simulink model "wheelchair_navigation"  (R2025b)
settings: Solver=VariableStepAuto  StartTime=0.0  StopTime=30  FixedStep=Ts  MaxStep=1.0  RelTol=1e-3
model workspace: external: MAT-File (data not in the file)
values from neighbouring files (symbols this model uses):
  a_max = 0.20    (= 0.2)    [init.m]
  AMCL_param = [rho,m_pos,q_pos,m_theta,q_theta,sigma_min_fact,sigma_max_fact,     p_fail,lost_duration,qt_lost_thd,max_jump_dist]    [init.m]
  d = 0.650    (= 0.65)    [init.m]
  e = 0.1    [init.m]
  epsilon = 0.5    [init.m]
  N = 20    [init.m]
  N_samples = 40    [init.m]
  omega_M = v_max/Rw    (= 1.52777777778)    [init.m]
  omega_m = -v_max/Rw    (= -1.52777777778)    [init.m]
  pos_estim_param = [sigma_q,sigma_m]    [init.m]
  q = 1    [init.m]
  r = 1    [init.m]
  r_c = 0.75    [init.m]
  r_red = 0.3    [init.m]
  Rw = 0.36    [init.m]
  s = (q+k^2*r)/(1-(1+Ts*k)^2)    (= 9.66666666667)    [init.m]
  sa = 10^3    (= 1000)    [init.m]
  sp = 10^9    (= 1000000000)    [init.m]
  T_gp = 4    [init.m]
  Ts = 0.2    [init.m]
  Ts_pedpos_est = 0.1    [init.m]
  v_max = 0.55    [init.m]
  x_p0 = startLoc(1)    [init.m]
  y_p0 = startLoc(2)    [init.m]
undefined symbols (not defined in the file or in its folder): endLoc, initial_cond, n_obs, param, Ped_init, qd, qdd, v_ped, v_ped_fun, x_pri, y_pri
libraries: simulink x1
settings Model: PacingRate=5  Creator=Lenovo ThinkPad  LastModifiedBy=bascetta
settings SolverCC: AlgebraicLoopSolver=TrustRegion
settings DataIOCC: SaveOutput=off  SignalLogging=off  DSMLogging=off  SaveTime=off  ReturnWorkspaceOutputs=off
settings OptimizationCC: ReuseModelBlockBuffer=off
settings DebuggingCC: UnconnectedInputMsg=warning  UnconnectedOutputMsg=warning  UnconnectedLineMsg=warning  UnderSpecifiedDimensionMsg=warning
settings ModelReferenceCC: EnableRefExpFcnMdlSchedulingChecks=on
settings SFSimCC: CustomCodeUndefinedFunction=UseInterfaceOnly
settings RTWCC: GPUComputeCapability=3.5  DLArmComputeVersion=19.05

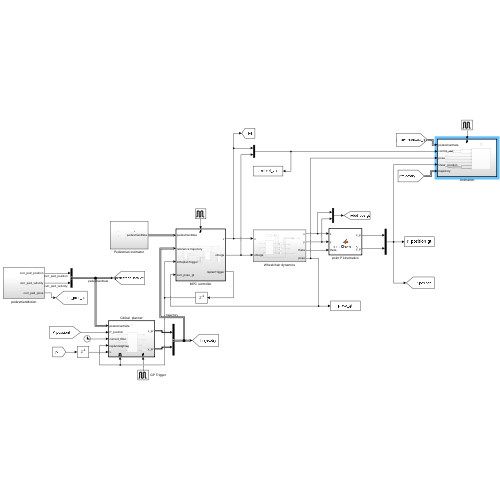
[thumbnail: Simulink's stored preview of the top-level diagram]
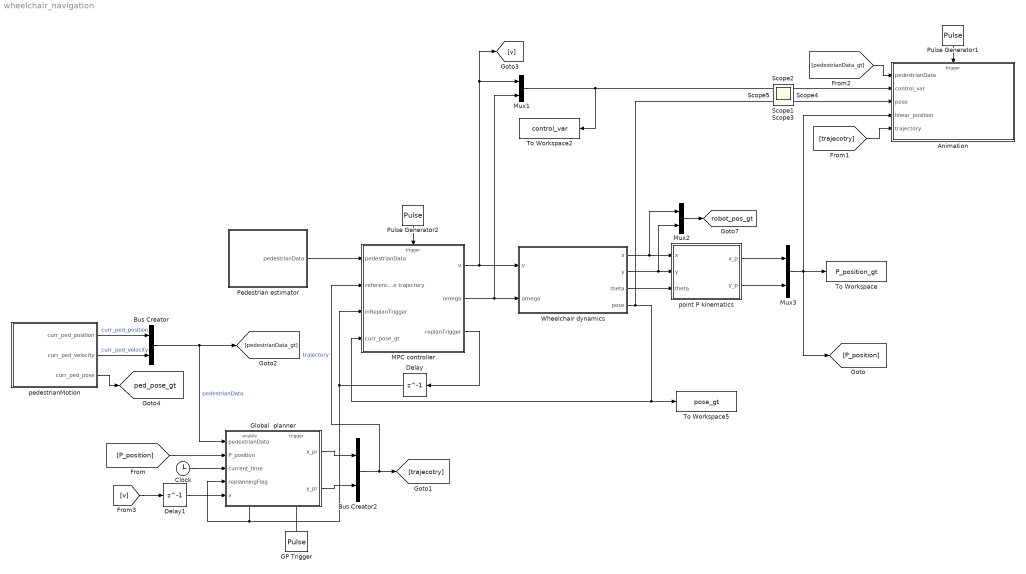
== system wheelchair_navigation ==
  Animation : Subsystem
  Bus Creator : BusCreator  Inputs=2
  Bus Creator2 : BusCreator  Inputs=2
  Clock : Clock
  Delay : Delay  DelayLength=1  InitialCondition=1  SampleTime=Ts
  Delay1 : Delay  DelayLength=1  InitialCondition=0  SampleTime=Ts
  GP Trigger : DiscretePulseGenerator  PulseType=Time based  Period=T_gp  PulseWidth=50  PhaseDelay=1e-16
  Global  planner : Subsystem
  MPC controller : Subsystem  TreatAsAtomicUnit=on
  Mux1 : Mux  Inputs=2
  Mux2 : Mux  Inputs=2
  Mux3 : Mux  Inputs=2
  Pedestrian estimator : Subsystem
  Pulse Generator1 : DiscretePulseGenerator  PulseType=Time based  Period=Ts  PulseWidth=50  PhaseDelay=1e-16
  Pulse Generator2 : DiscretePulseGenerator  PulseType=Time based  Period=Ts  PulseWidth=50  PhaseDelay=1e-16
  To Workspace : ToWorkspace  VariableName=P_position_gt  SaveFormat=Structure With Time  SampleTime=Ts
  To Workspace2 : ToWorkspace  VariableName=control_var  SaveFormat=Structure With Time  SampleTime=Ts
  To Workspace5 : ToWorkspace  VariableName=pose_gt  SaveFormat=Structure With Time  SampleTime=Ts
  "Wheelchair dynamics " : Subsystem
  pedestrianMotion : Subsystem
  point P kinematics : MATLAB Function  TreatAsAtomicUnit=on
  Scope{1..5} (5 alike) : Scope
      Scope1 settings: ActiveDisplayYMinimum=-0.0525  ActiveDisplayYMaximum=0.4725  DataLoggingVariableName=ScopeData3
      Scope3 settings: ActiveDisplayYMinimum=-0.13667  ActiveDisplayYMaximum=1.23002  DataLoggingVariableName=ScopeData2
      Scope5 settings: DataLoggingVariableName=ScopeData2
  tag scope: ped_pose_gt=global, robot_pos_gt=global
  wires:
  Pulse Generator2/1 -> MPC controller/Trigger
  "Wheelchair dynamics "/1(x) -> Mux2/1, point P kinematics/1(x)
  "Wheelchair dynamics "/2(y) -> Mux2/2, point P kinematics/2(y)
  "Wheelchair dynamics "/3(theta) -> point P kinematics/3(theta)
  MPC controller/1(v) -> [v], Mux1/1, "Wheelchair dynamics "/1(v)
  MPC controller/2(omega) -> Mux1/2, "Wheelchair dynamics "/2(omega)
  Mux1/1 -> To Workspace2/1, Animation/2(control_var)
  point P kinematics/1(x_p) -> Mux3/1
  point P kinematics/2(y_p) -> Mux3/2
  Pulse Generator1/1 -> Animation/Trigger
  Bus Creator/1 -> [pedestrianData_gt], Global  planner/1(pedestrianData)  "pedestrianData"
  pedestrianMotion/2(curr_ped_velocity) -> Bus Creator/2  "curr_ped_velocity"
  pedestrianMotion/1(curr_ped_position) -> Bus Creator/1  "curr_ped_position"
  [P_position] -> Global  planner/2(P_position)
  Clock/1 -> Global  planner/3(current_time)
  Global  planner/1(x_pr) -> Bus Creator2/1
  Global  planner/2(y_pr) -> Bus Creator2/2
  Bus Creator2/1 -> MPC controller/2(reference trajectory), [trajecotry]  "trajectory"
  [trajecotry] -> Animation/5(trajectory)
  [pedestrianData_gt] -> Animation/1(pedestrianData)
  MPC controller/3(replanTrigger) -> Delay/1
  Delay/1 -> Global  planner/4(replanningFlag), Global  planner/Enable, MPC controller/3(inReplanTrigger)
  Mux3/1 -> Animation/4(linear_position), To Workspace/1, [P_position]
  GP Trigger/1 -> Global  planner/Trigger
  [v] -> Delay1/1
  Delay1/1 -> Global  planner/5(v)
  pedestrianMotion/3(curr_ped_pose) -> [ped_pose_gt]
  Mux2/1 -> [robot_pos_gt]
  Pedestrian estimator/1(pedestrianData) -> MPC controller/1(pedestrianData)
  "Wheelchair dynamics "/4(pose) -> Animation/3(pose), To Workspace5/1, MPC controller/4("curr_pose_gt ")

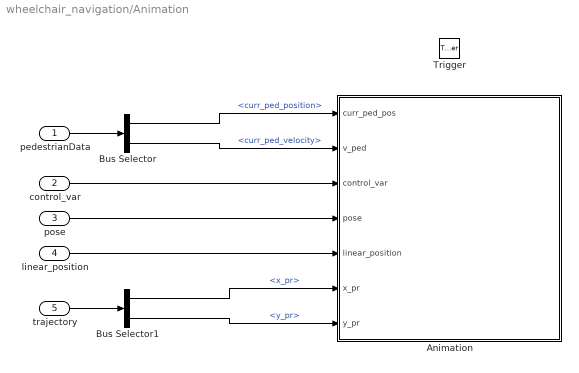
== system wheelchair_navigation/Animation ==
  pedestrianData : Inport
  control_var : Inport  Port=2
  pose : Inport  Port=3
  linear_position : Inport  Port=4
  trajectory : Inport  Port=5
  Trigger : TriggerPort  VariantControl=Variant  PortDimensions=1
  "Animation " : MATLAB Function  TreatAsAtomicUnit=on
  Bus Selector : BusSelector  OutputSignals=curr_ped_position,curr_ped_velocity
  Bus Selector1 : BusSelector  OutputSignals=x_pr,y_pr
  wires:
  pose/1 -> "Animation "/4(pose)
  control_var/1 -> "Animation "/3(control_var)
  linear_position/1 -> "Animation "/5(linear_position)
  pedestrianData/1 -> Bus Selector/1
  Bus Selector/1 -> "Animation "/1(curr_ped_pos)  "<curr_ped_position>"
  Bus Selector/2 -> "Animation "/2(v_ped)  "<curr_ped_velocity>"
  trajectory/1 -> Bus Selector1/1
  Bus Selector1/1 -> "Animation "/6(x_pr)  "<x_pr>"
  Bus Selector1/2 -> "Animation "/7(y_pr)  "<y_pr>"

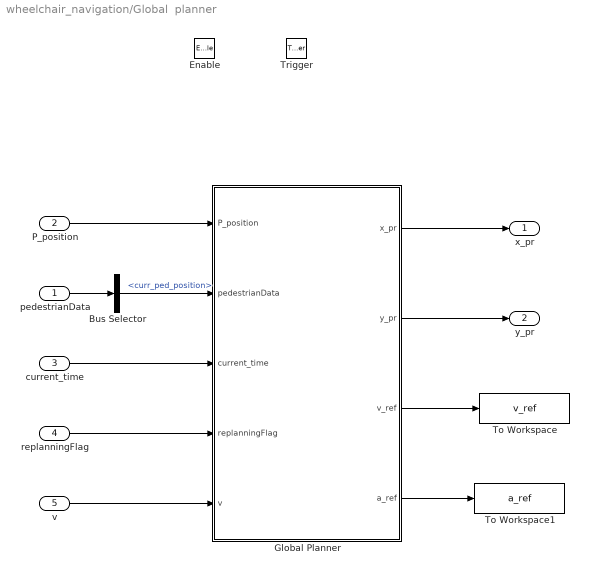
== system wheelchair_navigation/Global  planner ==
  pedestrianData : Inport
  P_position : Inport  Port=2
  current_time : Inport  Port=3
  replanningFlag : Inport  Port=4
  v : Inport  Port=5
  Enable : EnablePort  PropagateVarSize=During execution
  Trigger : TriggerPort  VariantControl=(inherit)  PortDimensions=1
  Bus Selector : BusSelector  OutputSignals=curr_ped_position
  Global Planner : MATLAB Function  TreatAsAtomicUnit=on
  To Workspace : ToWorkspace  VariableName=v_ref  SaveFormat=Timeseries  SampleTime=-1
  To Workspace1 : ToWorkspace  VariableName=a_ref  SaveFormat=Timeseries  SampleTime=-1
  x_pr : Outport
  y_pr : Outport  Port=2
  wires:
  current_time/1 -> Global Planner/3(current_time)
  Bus Selector/1 -> Global Planner/2(pedestrianData)  "<curr_ped_position>"
  pedestrianData/1 -> Bus Selector/1
  Global Planner/1(x_pr) -> x_pr/1
  Global Planner/2(y_pr) -> y_pr/1
  P_position/1 -> Global Planner/1(P_position)
  replanningFlag/1 -> Global Planner/4(replanningFlag)
  v/1 -> Global Planner/5(v)
  Global Planner/3(v_ref) -> To Workspace/1
  Global Planner/4(a_ref) -> To Workspace1/1

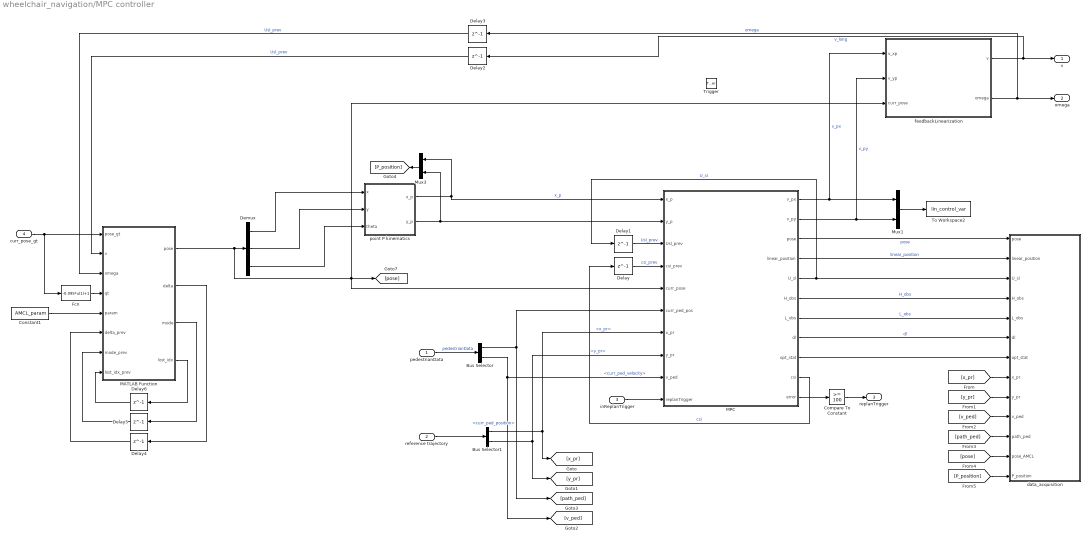
== system wheelchair_navigation/MPC controller ==
  pedestrianData : Inport
  reference trajectory : Inport  Port=2
  inReplanTrigger : Inport  Port=3
  "curr_pose_gt " : Inport  Port=4
  Trigger : TriggerPort  VariantControl=Variant
  Bus Selector : BusSelector  OutputSignals=curr_ped_position,curr_ped_velocity
  Bus Selector1 : BusSelector  OutputSignals=x_pr,y_pr
  Compare To Constant : simulink/Logic and Bit Operations/Compare To Constant  relop=>=  const=100  OutDataTypeStr=boolean
  Constant1 : Constant  Value=AMCL_param
  Delay : Delay  DelayLength=1  InitialCondition=[x_p0;y_p0]
  Delay1 : Delay  DelayLength=1  InitialCondition=0
  Delay2 : Delay  DelayLength=1  InitialCondition=0
  Delay3 : Delay  DelayLength=1  InitialCondition=0
  Delay4 : Delay  DelayLength=1
  Delay5 : Delay  DelayLength=1  InitialCondition=1.0
  Delay6 : Delay  DelayLength=1  InitialCondition=1.0
  Demux : Demux  Outputs=3
  Fcn : Fcn  Expr=-0.095*u(1)+1
  MATLAB Function : MATLAB Function  TreatAsAtomicUnit=on
  MPC : MATLAB Function  TreatAsAtomicUnit=on  mask{Ts=Ts, N=N, v_max=v_max, a_max=a_max, q=q, r=r, d=d, radius=Rw, max_omega=omega_M, min_omega=omega_m, epsilon=epsilon, n_obs=n_obs, e=e, N_samples=N_samples}
  Mux1 : Mux  Inputs=2
  Mux3 : Mux  Inputs=2
  To Workspace2 : ToWorkspace  VariableName=lin_control_var  SaveFormat=Structure With Time  SampleTime=-1
  data_acquisition : Subsystem
  feedbackLinearization : MATLAB Function  TreatAsAtomicUnit=on
  point P kinematics : MATLAB Function  TreatAsAtomicUnit=on
  v : Outport
  omega : Outport  Port=2
  replanTrigger : Outport  Port=3
  wires:
  Delay1/1 -> MPC/3(Usl_prev)  "Usl_prev"
  Delay/1 -> MPC/4(csi_prev)  "csi_prev"
  MPC/3(pose) -> data_acquisition/1(pose)  "pose"
  MPC/4(linear_position) -> data_acquisition/2(linear_position)  "linear_position"
  MPC/5(U_sl) -> Delay1/1, data_acquisition/3(U_sl)  "U_sl"
  MPC/6(H_obs) -> data_acquisition/4("H_obs ")  "H_obs"
  MPC/7(L_obs) -> data_acquisition/5("L_obs ")  "L_obs"
  MPC/8(dl) -> data_acquisition/6(dl)  "dl"
  MPC/10(csi) -> Delay/1  "csi"
  MPC/9(opt_stat) -> data_acquisition/7(opt_stat)
  MPC/1(v_px) -> Mux1/1, feedbackLinearization/1(v_xp)  "v_px"
  MPC/2(v_py) -> Mux1/2, feedbackLinearization/2(v_yp)  "v_py"
  Bus Selector/2 -> [v_ped], MPC/9(v_ped)  "<curr_ped_velocity>"
  pedestrianData/1 -> Bus Selector/1  "pedestrianData"
  Bus Selector/1 -> [path_ped], MPC/6(curr_ped_pos)  "<curr_ped_position>"
  Bus Selector1/1 -> [x_pr], MPC/7(x_pr)  "<x_pr>"
  Bus Selector1/2 -> [y_pr], MPC/8(y_pr)  "<y_pr>"
  reference trajectory/1 -> Bus Selector1/1
  MPC/11(error) -> Compare To Constant/1
  Compare To Constant/1 -> replanTrigger/1
  inReplanTrigger/1 -> MPC/10(replanTrigger)
  [x_pr] -> data_acquisition/8(x_pr)
  [y_pr] -> data_acquisition/9(y_pr)
  [v_ped] -> data_acquisition/10(v_ped)
  [path_ped] -> data_acquisition/11(path_ped)
  MATLAB Function/1(pose) -> MPC/5(curr_pose), feedbackLinearization/3(curr_pose), [pose], Demux/1
  Delay5/1 -> MATLAB Function/7(mode_prev)
  Demux/3 -> point P kinematics/3(theta)
  Delay2/1 -> MATLAB Function/2(v)  "Usl_prev"
  MATLAB Function/4(lost_idx) -> Delay6/1
  MATLAB Function/2(delta) -> Delay4/1
  MATLAB Function/3(mode) -> Delay5/1
  Constant1/1 -> MATLAB Function/5(param)
  Demux/2 -> point P kinematics/2(y)
  "curr_pose_gt "/1 -> Fcn/1, MATLAB Function/1(pose_gt)
  Delay6/1 -> MATLAB Function/8(lost_idx_prev)
  Demux/1 -> point P kinematics/1(x)
  Delay4/1 -> MATLAB Function/6(delta_prev)
  Delay3/1 -> MATLAB Function/3(omega)  "Usl_prev"
  Mux3/1 -> [P_position]
  point P kinematics/2(y_p) -> MPC/2(y_p), Mux3/2
  point P kinematics/1(x_p) -> MPC/1(x_p), Mux3/1  "x_p"
  feedbackLinearization/1(v) -> Delay2/1, v/1  "v_long"
  feedbackLinearization/2(omega) -> Delay3/1, omega/1  "omega"
  [pose] -> data_acquisition/12(pose_AMCL)
  [P_position] -> data_acquisition/13(P_position)
  Fcn/1 -> MATLAB Function/4(qt)
  Mux1/1 -> To Workspace2/1

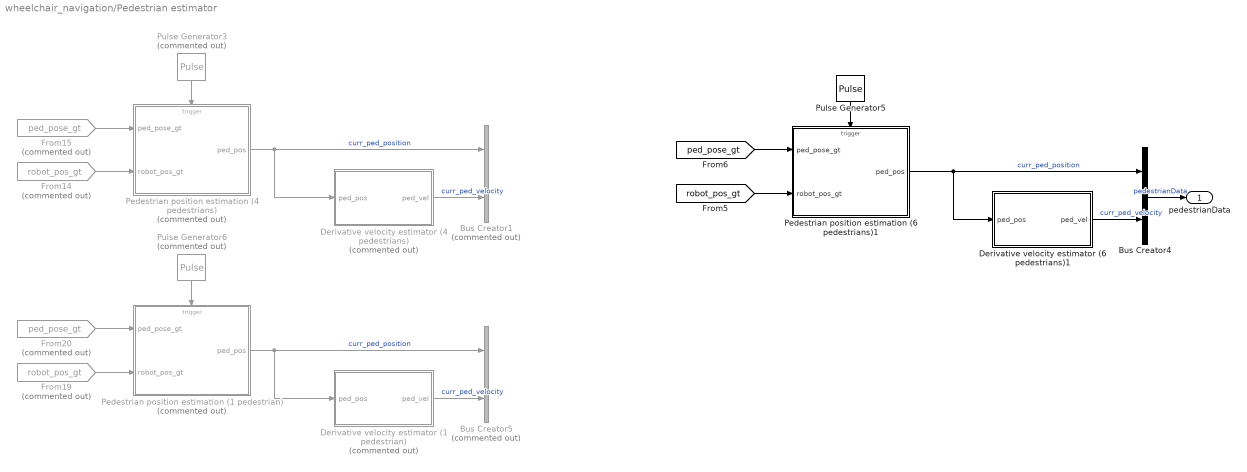
== system wheelchair_navigation/Pedestrian estimator ==
  Bus Creator1 : BusCreator  Commented=on  Inputs=2
  Bus Creator4 : BusCreator  Inputs=2
  Bus Creator5 : BusCreator  Commented=on  Inputs=2
  Derivative velocity estimator (1 pedestrian) : Subsystem  Commented=on
  Derivative velocity estimator (4 pedestrians) : Subsystem  Commented=on
  Derivative velocity estimator (6 pedestrians)1 : Subsystem
  From14 : From  Commented=on  GotoTag=robot_pos_gt
  From15 : From  Commented=on  GotoTag=ped_pose_gt
  From19 : From  Commented=on  GotoTag=robot_pos_gt  TagVisibility=global
  From20 : From  Commented=on  GotoTag=ped_pose_gt  TagVisibility=global
  Pedestrian position estimation (1 pedestrian) : Subsystem  Commented=on  TreatAsAtomicUnit=on
  Pedestrian position estimation (4 pedestrians) : Subsystem  Commented=on  TreatAsAtomicUnit=on
  Pedestrian position estimation (6 pedestrians)1 : Subsystem  TreatAsAtomicUnit=on
  Pulse Generator3 : DiscretePulseGenerator  Commented=on  PulseType=Time based  Period=Ts_pedpos_est  PulseWidth=50  PhaseDelay=1e-16
  Pulse Generator5 : DiscretePulseGenerator  PulseType=Time based  Period=Ts_pedpos_est  PulseWidth=50  PhaseDelay=1e-16
  Pulse Generator6 : DiscretePulseGenerator  Commented=on  PulseType=Time based  Period=Ts_pedpos_est  PulseWidth=50  PhaseDelay=1e-16
  pedestrianData : Outport
  wires:
  Pedestrian position estimation (1 pedestrian)/1(ped_pos) -> Derivative velocity estimator (1 pedestrian)/1(ped_pos), Bus Creator5/1  "curr_ped_position"
  [robot_pos_gt] -> Pedestrian position estimation (6 pedestrians)1/2(robot_pos_gt)
  Derivative velocity estimator (1 pedestrian)/1(ped_vel) -> Bus Creator5/2  "curr_ped_velocity"
  From19/1 -> Pedestrian position estimation (1 pedestrian)/2(robot_pos_gt)
  From14/1 -> Pedestrian position estimation (4 pedestrians)/2(robot_pos_gt)
  From15/1 -> Pedestrian position estimation (4 pedestrians)/1(ped_pose_gt)
  [ped_pose_gt] -> Pedestrian position estimation (6 pedestrians)1/1(ped_pose_gt)
  Derivative velocity estimator (6 pedestrians)1/1(ped_vel) -> Bus Creator4/2  "curr_ped_velocity"
  Pulse Generator5/1 -> Pedestrian position estimation (6 pedestrians)1/Trigger
  Pulse Generator3/1 -> Pedestrian position estimation (4 pedestrians)/Trigger
  From20/1 -> Pedestrian position estimation (1 pedestrian)/1(ped_pose_gt)
  Pulse Generator6/1 -> Pedestrian position estimation (1 pedestrian)/Trigger
  Derivative velocity estimator (4 pedestrians)/1(ped_vel) -> Bus Creator1/2  "curr_ped_velocity"
  Pedestrian position estimation (4 pedestrians)/1(ped_pos) -> Derivative velocity estimator (4 pedestrians)/1(ped_pos), Bus Creator1/1  "curr_ped_position"
  Pedestrian position estimation (6 pedestrians)1/1(ped_pos) -> Derivative velocity estimator (6 pedestrians)1/1(ped_pos), Bus Creator4/1  "curr_ped_position"
  Bus Creator4/1 -> pedestrianData/1  "pedestrianData"

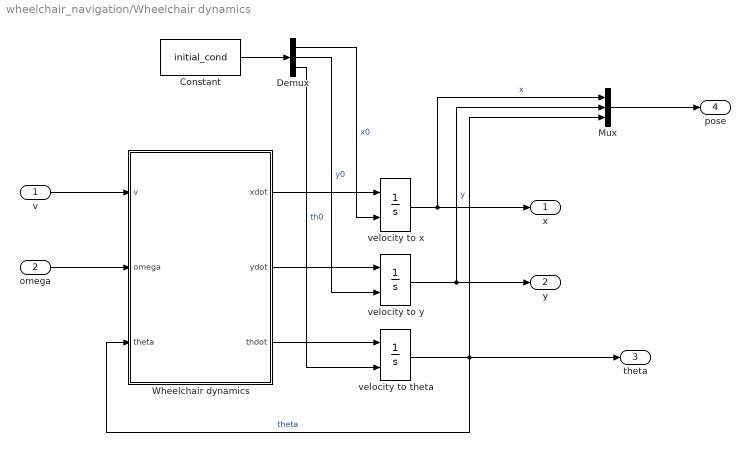
== system wheelchair_navigation/Wheelchair dynamics  ==
  v : Inport
  omega : Inport  Port=2
  Constant : Constant  Value=initial_cond
  Demux : Demux  Outputs=3
  Mux : Mux  Inputs=3
  "Wheelchair dynamics " : MATLAB Function  TreatAsAtomicUnit=on
  velocity to theta : Integrator  InitialConditionSource=external
  velocity to x : Integrator  InitialConditionSource=external
  velocity to y : Integrator  InitialConditionSource=external
  x : Outport
  y : Outport  Port=2
  theta : Outport  Port=3
  pose : Outport  Port=4
  wires:
  omega/1 -> "Wheelchair dynamics "/2(omega)
  "Wheelchair dynamics "/1(xdot) -> velocity to x/1
  "Wheelchair dynamics "/3(thdot) -> velocity to theta/1
  v/1 -> "Wheelchair dynamics "/1(v)
  "Wheelchair dynamics "/2(ydot) -> velocity to y/1
  Mux/1 -> pose/1
  Demux/1 -> velocity to x/2  "x0"
  Demux/2 -> velocity to y/2  "y0"
  velocity to x/1 -> Mux/1, x/1  "x"
  velocity to y/1 -> Mux/2, y/1  "y"
  Demux/3 -> velocity to theta/2  "th0"
  Constant/1 -> Demux/1
  velocity to theta/1 -> theta/1, "Wheelchair dynamics "/3(theta), Mux/3  "theta"

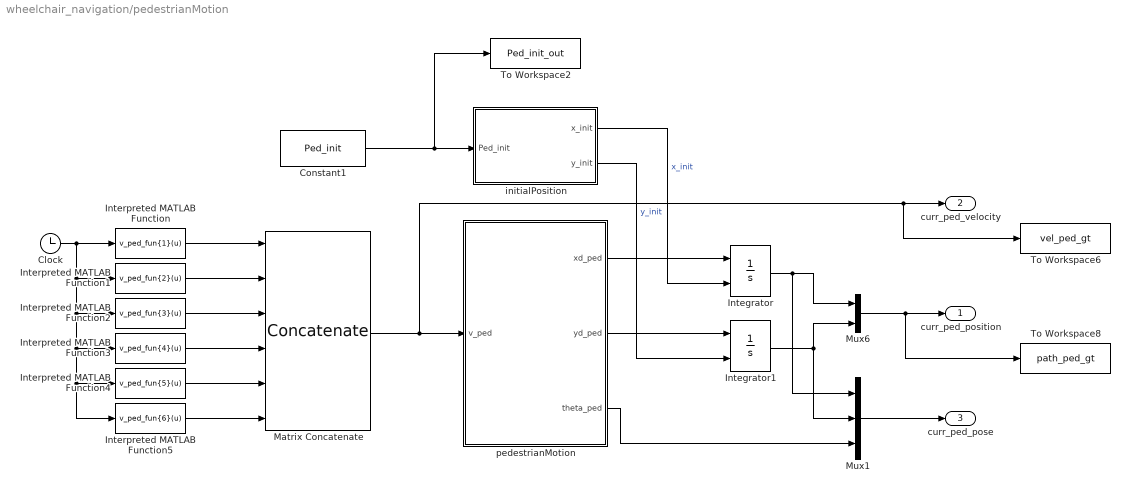
== system wheelchair_navigation/pedestrianMotion ==
  Clock : Clock
  Constant1 : Constant  Value=Ped_init  VectorParams1D=off
  Integrator : Integrator  InitialConditionSource=external
  Integrator1 : Integrator  InitialConditionSource=external
  Interpreted MATLAB Function : MATLABFcn  MATLABFcn=v_ped_fun{1}(u)  Output1D=off
  Interpreted MATLAB Function1 : MATLABFcn  MATLABFcn=v_ped_fun{2}(u)  Output1D=off
  Interpreted MATLAB Function2 : MATLABFcn  MATLABFcn=v_ped_fun{3}(u)  Output1D=off
  Interpreted MATLAB Function3 : MATLABFcn  MATLABFcn=v_ped_fun{4}(u)  Output1D=off
  Interpreted MATLAB Function4 : MATLABFcn  MATLABFcn=v_ped_fun{5}(u)  Output1D=off
  Interpreted MATLAB Function5 : MATLABFcn  MATLABFcn=v_ped_fun{6}(u)  Output1D=off
  Matrix Concatenate : Concatenate  NumInputs=6  Mode=Multidimensional array
  Mux1 : Mux  Inputs=3
  Mux6 : Mux  Inputs=2
  To Workspace2 : ToWorkspace  VariableName=Ped_init_out  SaveFormat=Timeseries  SampleTime=-1
  To Workspace6 : ToWorkspace  VariableName=vel_ped_gt  SaveFormat=Structure With Time  SampleTime=Ts
  To Workspace8 : ToWorkspace  VariableName=path_ped_gt  SaveFormat=Structure With Time  SampleTime=Ts
  initialPosition : MATLAB Function  TreatAsAtomicUnit=on
  pedestrianMotion : MATLAB Function  TreatAsAtomicUnit=on
  curr_ped_position : Outport
  curr_ped_velocity : Outport  Port=2
  curr_ped_pose : Outport  Port=3
  wires:
  pedestrianMotion/1(xd_ped) -> Integrator/1
  Integrator1/1 -> Mux6/2, Mux1/2
  Matrix Concatenate/1 -> To Workspace6/1, curr_ped_velocity/1, pedestrianMotion/1(v_ped)
  initialPosition/2(y_init) -> Integrator1/2  "y_init"
  initialPosition/1(x_init) -> Integrator/2  "x_init"
  Constant1/1 -> To Workspace2/1, initialPosition/1(Ped_init)
  Mux6/1 -> To Workspace8/1, curr_ped_position/1
  Mux1/1 -> curr_ped_pose/1
  Integrator/1 -> Mux1/1, Mux6/1
  pedestrianMotion/3(theta_ped) -> Mux1/3
  pedestrianMotion/2(yd_ped) -> Integrator1/1
  Interpreted MATLAB Function2/1 -> Matrix Concatenate/3
  Interpreted MATLAB Function3/1 -> Matrix Concatenate/4
  Interpreted MATLAB Function/1 -> Matrix Concatenate/1
  Interpreted MATLAB Function1/1 -> Matrix Concatenate/2
  Clock/1 -> Interpreted MATLAB Function5/1, Interpreted MATLAB Function4/1, Interpreted MATLAB Function3/1, Interpreted MATLAB Function2/1, Interpreted MATLAB Function1/1, Interpreted MATLAB Function/1
  Interpreted MATLAB Function4/1 -> Matrix Concatenate/5
  Interpreted MATLAB Function5/1 -> Matrix Concatenate/6

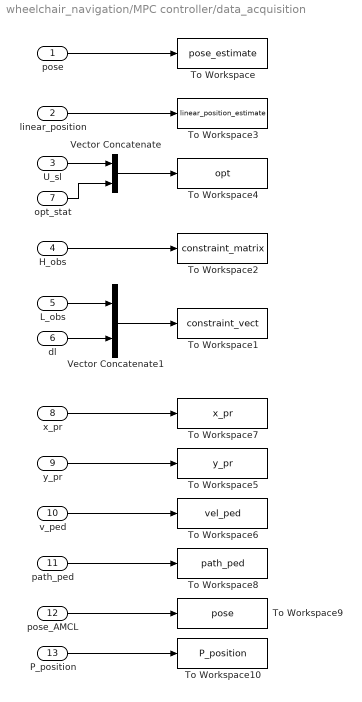
== system wheelchair_navigation/MPC controller/data_acquisition ==
  pose : Inport
  linear_position : Inport  Port=2
  U_sl : Inport  Port=3
  "H_obs " : Inport  Port=4
  "L_obs " : Inport  Port=5
  dl : Inport  Port=6
  opt_stat : Inport  Port=7
  x_pr : Inport  Port=8
  y_pr : Inport  Port=9
  v_ped : Inport  Port=10
  path_ped : Inport  Port=11
  pose_AMCL : Inport  Port=12
  P_position : Inport  Port=13
  To Workspace : ToWorkspace  VariableName=pose_estimate  SaveFormat=Structure  SampleTime=-1
  To Workspace1 : ToWorkspace  VariableName=constraint_vect  SaveFormat=Structure  SampleTime=-1
  To Workspace10 : ToWorkspace  VariableName=P_position  SaveFormat=Structure With Time  SampleTime=-1
  To Workspace2 : ToWorkspace  VariableName=constraint_matrix  SaveFormat=Structure  SampleTime=-1
  To Workspace3 : ToWorkspace  VariableName=linear_position_estimate  SaveFormat=Structure  SampleTime=-1
  To Workspace4 : ToWorkspace  VariableName=opt  SaveFormat=Structure With Time  SampleTime=-1
  To Workspace5 : ToWorkspace  VariableName=y_pr  SaveFormat=Structure With Time  SampleTime=-1
  To Workspace6 : ToWorkspace  VariableName=vel_ped  SaveFormat=Structure With Time  SampleTime=-1
  To Workspace7 : ToWorkspace  VariableName=x_pr  SaveFormat=Structure With Time  SampleTime=-1
  To Workspace8 : ToWorkspace  VariableName=path_ped  SaveFormat=Structure With Time  SampleTime=-1
  To Workspace9 : ToWorkspace  VariableName=pose  SaveFormat=Structure With Time  SampleTime=-1
  Vector Concatenate : Concatenate  ConcatenateDimension=2
  Vector Concatenate1 : Concatenate  Mode=Multidimensional array  ConcatenateDimension=2
  wires:
  "H_obs "/1 -> To Workspace2/1
  linear_position/1 -> To Workspace3/1
  pose/1 -> To Workspace/1
  "L_obs "/1 -> Vector Concatenate1/1
  dl/1 -> Vector Concatenate1/2
  Vector Concatenate1/1 -> To Workspace1/1
  U_sl/1 -> Vector Concatenate/1
  Vector Concatenate/1 -> To Workspace4/1
  opt_stat/1 -> Vector Concatenate/2
  x_pr/1 -> To Workspace7/1
  path_ped/1 -> To Workspace8/1
  v_ped/1 -> To Workspace6/1
  y_pr/1 -> To Workspace5/1
  P_position/1 -> To Workspace10/1
  pose_AMCL/1 -> To Workspace9/1

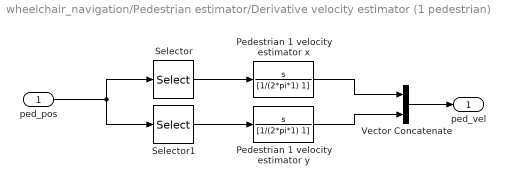
== system wheelchair_navigation/Pedestrian estimator/Derivative velocity estimator (1 pedestrian) ==
  ped_pos : Inport
  Pedestrian 1 velocity estimator x : TransferFcn  Numerator=[1 0]  Denominator=[1/(2*pi*1) 1]
  Pedestrian 1 velocity estimator y : TransferFcn  Numerator=[1 0]  Denominator=[1/(2*pi*1) 1]
  Selector : Selector  InputPortWidth=2  IndexOptions=Index vector (dialog)  Indices=[1]  OutputSizes=1
  Selector1 : Selector  InputPortWidth=2  IndexOptions=Index vector (dialog)  Indices=[2]  OutputSizes=1
  Vector Concatenate : Concatenate  Mode=Multidimensional array  ConcatenateDimension=2
  ped_vel : Outport
  wires:
  Vector Concatenate/1 -> ped_vel/1
  Selector/1 -> Pedestrian 1 velocity estimator x/1
  Selector1/1 -> Pedestrian 1 velocity estimator y/1
  ped_pos/1 -> Selector1/1, Selector/1
  Pedestrian 1 velocity estimator x/1 -> Vector Concatenate/1
  Pedestrian 1 velocity estimator y/1 -> Vector Concatenate/2

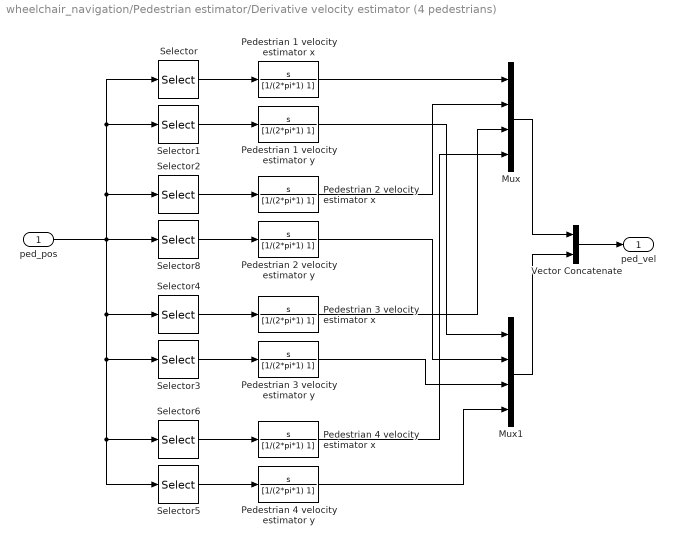
== system wheelchair_navigation/Pedestrian estimator/Derivative velocity estimator (4 pedestrians) ==
  ped_pos : Inport
  Mux : Mux
  Mux1 : Mux
  Pedestrian 1 velocity estimator x : TransferFcn  Numerator=[1 0]  Denominator=[1/(2*pi*1) 1]
  Pedestrian 1 velocity estimator y : TransferFcn  Numerator=[1 0]  Denominator=[1/(2*pi*1) 1]
  Pedestrian 2 velocity estimator x : TransferFcn  Numerator=[1 0]  Denominator=[1/(2*pi*1) 1]
  Pedestrian 2 velocity estimator y : TransferFcn  Numerator=[1 0]  Denominator=[1/(2*pi*1) 1]
  Pedestrian 3 velocity estimator x : TransferFcn  Numerator=[1 0]  Denominator=[1/(2*pi*1) 1]
  Pedestrian 3 velocity estimator y : TransferFcn  Numerator=[1 0]  Denominator=[1/(2*pi*1) 1]
  Pedestrian 4 velocity estimator x : TransferFcn  Numerator=[1 0]  Denominator=[1/(2*pi*1) 1]
  Pedestrian 4 velocity estimator y : TransferFcn  Numerator=[1 0]  Denominator=[1/(2*pi*1) 1]
  Selector : Selector  InputPortWidth=8  IndexOptions=Index vector (dialog)  Indices=[1]  OutputSizes=1
  Selector1 : Selector  InputPortWidth=8  IndexOptions=Index vector (dialog)  Indices=[5]  OutputSizes=1
  Selector2 : Selector  InputPortWidth=8  IndexOptions=Index vector (dialog)  Indices=[2]  OutputSizes=1
  Selector3 : Selector  InputPortWidth=8  IndexOptions=Index vector (dialog)  Indices=[7]  OutputSizes=1
  Selector4 : Selector  InputPortWidth=8  IndexOptions=Index vector (dialog)  Indices=[3]  OutputSizes=1
  Selector5 : Selector  InputPortWidth=8  IndexOptions=Index vector (dialog)  Indices=[8]  OutputSizes=1
  Selector6 : Selector  InputPortWidth=8  IndexOptions=Index vector (dialog)  Indices=[4]  OutputSizes=1
  Selector8 : Selector  InputPortWidth=8  IndexOptions=Index vector (dialog)  Indices=[6]  OutputSizes=1
  Vector Concatenate : Concatenate  Mode=Multidimensional array  ConcatenateDimension=2
  ped_vel : Outport
  wires:
  Vector Concatenate/1 -> ped_vel/1
  Mux1/1 -> Vector Concatenate/2
  Mux/1 -> Vector Concatenate/1
  Pedestrian 1 velocity estimator y/1 -> Mux1/1
  Pedestrian 2 velocity estimator x/1 -> Mux/2
  Pedestrian 3 velocity estimator y/1 -> Mux1/3
  Pedestrian 4 velocity estimator y/1 -> Mux1/4
  Pedestrian 4 velocity estimator x/1 -> Mux/4
  Pedestrian 3 velocity estimator x/1 -> Mux/3
  Pedestrian 1 velocity estimator x/1 -> Mux/1
  Selector6/1 -> Pedestrian 4 velocity estimator x/1
  Selector4/1 -> Pedestrian 3 velocity estimator x/1
  Selector2/1 -> Pedestrian 2 velocity estimator x/1
  ped_pos/1 -> Selector8/1, Selector1/1, Selector/1, Selector2/1, Selector3/1, Selector5/1, Selector6/1, Selector4/1
  Selector/1 -> Pedestrian 1 velocity estimator x/1
  Selector1/1 -> Pedestrian 1 velocity estimator y/1
  Pedestrian 2 velocity estimator y/1 -> Mux1/2
  Selector8/1 -> Pedestrian 2 velocity estimator y/1
  Selector3/1 -> Pedestrian 3 velocity estimator y/1
  Selector5/1 -> Pedestrian 4 velocity estimator y/1

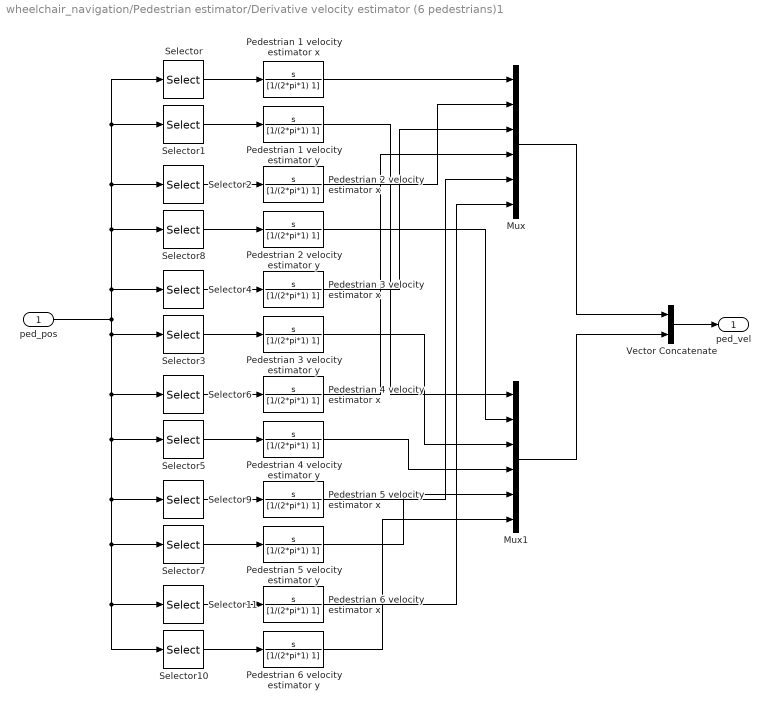
== system wheelchair_navigation/Pedestrian estimator/Derivative velocity estimator (6 pedestrians)1 ==
  ped_pos : Inport
  Mux : Mux  Inputs=6
  Mux1 : Mux  Inputs=6
  Pedestrian 1 velocity estimator x : TransferFcn  Numerator=[1 0]  Denominator=[1/(2*pi*1) 1]
  Pedestrian 1 velocity estimator y : TransferFcn  Numerator=[1 0]  Denominator=[1/(2*pi*1) 1]
  Pedestrian 2 velocity estimator x : TransferFcn  Numerator=[1 0]  Denominator=[1/(2*pi*1) 1]
  Pedestrian 2 velocity estimator y : TransferFcn  Numerator=[1 0]  Denominator=[1/(2*pi*1) 1]
  Pedestrian 3 velocity estimator x : TransferFcn  Numerator=[1 0]  Denominator=[1/(2*pi*1) 1]
  Pedestrian 3 velocity estimator y : TransferFcn  Numerator=[1 0]  Denominator=[1/(2*pi*1) 1]
  Pedestrian 4 velocity estimator x : TransferFcn  Numerator=[1 0]  Denominator=[1/(2*pi*1) 1]
  Pedestrian 4 velocity estimator y : TransferFcn  Numerator=[1 0]  Denominator=[1/(2*pi*1) 1]
  Pedestrian 5 velocity estimator x : TransferFcn  Numerator=[1 0]  Denominator=[1/(2*pi*1) 1]
  Pedestrian 5 velocity estimator y : TransferFcn  Numerator=[1 0]  Denominator=[1/(2*pi*1) 1]
  Pedestrian 6 velocity estimator x : TransferFcn  Numerator=[1 0]  Denominator=[1/(2*pi*1) 1]
  Pedestrian 6 velocity estimator y : TransferFcn  Numerator=[1 0]  Denominator=[1/(2*pi*1) 1]
  Selector : Selector  InputPortWidth=12  IndexOptions=Index vector (dialog)  Indices=[1]  OutputSizes=1
  Selector1 : Selector  InputPortWidth=12  IndexOptions=Index vector (dialog)  Indices=[7]  OutputSizes=1
  Selector10 : Selector  InputPortWidth=12  IndexOptions=Index vector (dialog)  Indices=[12]  OutputSizes=1
  Selector11 : Selector  InputPortWidth=12  IndexOptions=Index vector (dialog)  Indices=[6]  OutputSizes=1
  Selector2 : Selector  InputPortWidth=12  IndexOptions=Index vector (dialog)  Indices=[2]  OutputSizes=1
  Selector3 : Selector  InputPortWidth=12  IndexOptions=Index vector (dialog)  Indices=[9]  OutputSizes=1
  Selector4 : Selector  InputPortWidth=12  IndexOptions=Index vector (dialog)  Indices=[3]  OutputSizes=1
  Selector5 : Selector  InputPortWidth=12  IndexOptions=Index vector (dialog)  Indices=[10]  OutputSizes=1
  Selector6 : Selector  InputPortWidth=12  IndexOptions=Index vector (dialog)  Indices=[4]  OutputSizes=1
  Selector7 : Selector  InputPortWidth=12  IndexOptions=Index vector (dialog)  Indices=[11]  OutputSizes=1
  Selector8 : Selector  InputPortWidth=12  IndexOptions=Index vector (dialog)  Indices=[8]  OutputSizes=1
  Selector9 : Selector  InputPortWidth=12  IndexOptions=Index vector (dialog)  Indices=[5]  OutputSizes=1
  Vector Concatenate : Concatenate  Mode=Multidimensional array  ConcatenateDimension=2
  ped_vel : Outport
  wires:
  Vector Concatenate/1 -> ped_vel/1
  Selector4/1 -> Pedestrian 3 velocity estimator x/1
  Selector3/1 -> Pedestrian 3 velocity estimator y/1
  ped_pos/1 -> Selector10/1, Selector11/1, Selector7/1, Selector9/1, Selector5/1, Selector6/1, Selector3/1, Selector8/1, Selector1/1, Selector/1, Selector2/1, Selector4/1
  Selector/1 -> Pedestrian 1 velocity estimator x/1
  Selector1/1 -> Pedestrian 1 velocity estimator y/1
  Selector6/1 -> Pedestrian 4 velocity estimator x/1
  Selector8/1 -> Pedestrian 2 velocity estimator y/1
  Selector5/1 -> Pedestrian 4 velocity estimator y/1
  Selector2/1 -> Pedestrian 2 velocity estimator x/1
  Selector7/1 -> Pedestrian 5 velocity estimator y/1
  Selector9/1 -> Pedestrian 5 velocity estimator x/1
  Selector11/1 -> Pedestrian 6 velocity estimator x/1
  Selector10/1 -> Pedestrian 6 velocity estimator y/1
  Pedestrian 1 velocity estimator x/1 -> Mux/1
  Pedestrian 2 velocity estimator x/1 -> Mux/2
  Pedestrian 3 velocity estimator x/1 -> Mux/3
  Pedestrian 4 velocity estimator x/1 -> Mux/4
  Pedestrian 5 velocity estimator x/1 -> Mux/5
  Pedestrian 6 velocity estimator x/1 -> Mux/6
  Pedestrian 1 velocity estimator y/1 -> Mux1/1
  Pedestrian 2 velocity estimator y/1 -> Mux1/2
  Pedestrian 3 velocity estimator y/1 -> Mux1/3
  Pedestrian 4 velocity estimator y/1 -> Mux1/4
  Pedestrian 5 velocity estimator y/1 -> Mux1/5
  Pedestrian 6 velocity estimator y/1 -> Mux1/6
  Mux/1 -> Vector Concatenate/1
  Mux1/1 -> Vector Concatenate/2

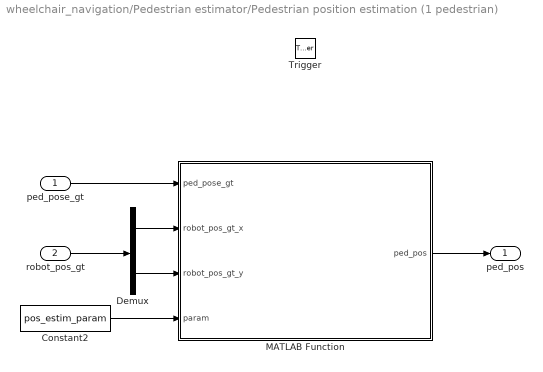
== system wheelchair_navigation/Pedestrian estimator/Pedestrian position estimation (1 pedestrian) ==
  ped_pose_gt : Inport
  robot_pos_gt : Inport  Port=2
  Trigger : TriggerPort  VariantControl=(inherit)
  Constant2 : Constant  Value=pos_estim_param
  Demux : Demux  Outputs=2
  MATLAB Function : MATLAB Function  TreatAsAtomicUnit=on
  ped_pos : Outport
  wires:
  Constant2/1 -> MATLAB Function/4(param)
  MATLAB Function/1(ped_pos) -> ped_pos/1
  ped_pose_gt/1 -> MATLAB Function/1(ped_pose_gt)
  Demux/2 -> MATLAB Function/3(robot_pos_gt_y)
  Demux/1 -> MATLAB Function/2(robot_pos_gt_x)
  robot_pos_gt/1 -> Demux/1

== system wheelchair_navigation/Pedestrian estimator/Pedestrian position estimation (4 pedestrians) ==
  ped_pose_gt : Inport
  robot_pos_gt : Inport  Port=2
  Trigger : TriggerPort  VariantControl=(inherit)
  Constant2 : Constant  Value=pos_estim_param
  Demux : Demux  Outputs=2
  MATLAB Function : MATLAB Function  TreatAsAtomicUnit=on
  ped_pos : Outport
  wires:
  Constant2/1 -> MATLAB Function/4(param)
  MATLAB Function/1(ped_pos) -> ped_pos/1
  ped_pose_gt/1 -> MATLAB Function/1(ped_pose_gt)
  Demux/2 -> MATLAB Function/3(robot_pos_gt_y)
  Demux/1 -> MATLAB Function/2(robot_pos_gt_x)
  robot_pos_gt/1 -> Demux/1

== system wheelchair_navigation/Pedestrian estimator/Pedestrian position estimation (6 pedestrians)1 ==
  ped_pose_gt : Inport
  robot_pos_gt : Inport  Port=2
  Trigger : TriggerPort  VariantControl=(inherit)
  Constant2 : Constant  Value=pos_estim_param
  Demux : Demux  Outputs=2
  MATLAB Function : MATLAB Function  TreatAsAtomicUnit=on
  ped_pos : Outport
  wires:
  Constant2/1 -> MATLAB Function/4(param)
  MATLAB Function/1(ped_pos) -> ped_pos/1
  ped_pose_gt/1 -> MATLAB Function/1(ped_pose_gt)
  Demux/2 -> MATLAB Function/3(robot_pos_gt_y)
  Demux/1 -> MATLAB Function/2(robot_pos_gt_x)
  robot_pos_gt/1 -> Demux/1

== matlab function wheelchair_navigation/MPC controller/feedbackLinearization ==
  data: v_xp input; v_yp input; curr_pose input size=3; v output; omega output; epsilon parameter
function [v, omega]= feedbackLinearization(v_xp, v_yp, curr_pose, epsilon)
    
    theta = curr_pose(3);
    v = v_xp*cos(theta)+v_yp*sin(theta);
    omega = (v_yp*cos(theta)-v_xp*sin(theta))/epsilon;
    
end

== matlab function wheelchair_navigation/point P kinematics ==
  data: x input; x_p output; y input; theta input; y_p output; epsilon parameter
function [x_p,y_p] = pointKinematics(x,y,theta,epsilon)

    
    x_p = x+epsilon*cos(theta);
    y_p = y+epsilon*sin(theta);

end

== matlab function wheelchair_navigation/Animation/Animation  ==
  data: curr_ped_pos input; v_ped input; control_var input; pose input; linear_position input; x_pr input; y_pr input; epsilon parameter; x_p0 parameter; y_p0 parameter; n_obs parameter; r_red parameter; r_c parameter; endLoc parameter; param parameter
function animation(curr_ped_pos, v_ped, control_var, pose, linear_position, x_pr, y_pr, epsilon, x_p0, y_p0, n_obs, r_red, r_c, endLoc, param)

coder.extrinsic('scatter','quiver','mkdir');

%Robot pose
x = pose(1); y = pose(2); theta = pose(3);

%Robot linear Position
x_p=linear_position(1); y_p=linear_position(2);

persistent idx
if isempty(idx)
    idx = 0;
end

persistent check_dir
if isempty(check_dir)
    check_dir = 0;
end

persistent id_dir
if isempty(id_dir)
    id_dir = 0;
end

idx = idx + 1;
filename = sprintf('frame_%03d.png', int32(idx));


%Control variables
v = control_var(1);
omega = control_var(2);

%Transformation matrix
T = [cos(theta) -epsilon*sin(theta);
    sin(theta)  epsilon*cos(theta)];
vp_x = T(1,:)*[v; omega];
vp_y = T(2,:)*[v; omega];


% Struct to deal with multiple obstacle in the animation
obst=struct('PSf',zeros(2,6284),'VB',zeros(2,6284),'reducedVB',zeros(2,6284));
obst=repmat(obst,n_obs);

group=struct('hx', 0, 'hy', 0, 'l', 0,'Q1',zeros(2,1),'Q2',zeros(2,1));

%Pedestrian position
x_ped=zeros(n_obs,1); y_ped=zeros(n_obs,1);
x_ped(1:n_obs,1)=curr_ped_pos(1:n_obs);
y_ped(1:n_obs,1)=curr_ped_pos(n_obs+1:end);

% sensor Range drawings
th = 0:pi/50:2*pi;
xunit = param.sensorRange * cos(th) + x;
yunit = param.sensorRange * sin(th) + y;

if check_dir == 0
    while exist(sprintf('output/video_%d',int32(id_dir)),'dir')
        id_dir=id_dir+1;
    end
    check_dir=1;
end

%Initialization of vectors containing pedestrians predicted motion
current_x_ped = zeros(n_obs,1);
current_y_ped = zeros(n_obs,1);

%Position of pedestrians (obstacle) within the prediction horizon
current_x_ped(1:n_obs,1)=curr_ped_pos(1:n_obs);
current_y_ped(1:n_obs,1)=curr_ped_pos(n_obs+1:end);

X_ped = [current_x_ped, current_y_ped];

%index = dbscan(X_ped,2.7,1);

index = 1:1:n_obs;

n_groups = max(index);

group=repmat(group,n_groups);

x_plot=-10:0.1:20;

cla
hold on
for i_obs=1:n_obs
    %personal space function
    VR=[v*cos(theta)-v_ped(i_obs,1);
        v*sin(theta)-v_ped(i_obs,2)];

    %robot position P1
    P1=[x;y];

    %pedestrian position P2
    P2=[x_ped(i_obs);y_ped(i_obs)];
    [obst(i_obs).PSf,obst(i_obs).VB,obst(i_obs).reducedVB] = PsfData(P2,P1,VR,v_ped(i_obs,:),r_c,r_red);

    %plot pedestrians
    plot(obst(i_obs).PSf(1,:),obst(i_obs).PSf(2,:),'r');plot(obst(i_obs).VB(1,:),obst(i_obs).VB(2,:),'k');plot(obst(i_obs).reducedVB(1,:),obst(i_obs).reducedVB(2,:),'k');

end
VR=[v*cos(theta)-v_ped(:,1), v*sin(theta)-v_ped(:,2)];

%robot position P1
P1=[x;y];

%pedestrian position P2
P2=[x_ped, y_ped];

for i_obs=1:n_groups
    [group(i_obs).Q1,group(i_obs).Q2,robot_inside_obst]=findTangentPoints_convex_hull(P1, P2, v_ped, VR, r_c, r_red, index, i_obs, 50);
    %personal space function

    v1=[group(i_obs).Q1(1)-P1(1);
        group(i_obs).Q1(2)-P1(2)];
    v2=[group(i_obs).Q2(1)-P1(1);
        group(i_obs).Q2(2)-P1(2)];
    V_12=[v1 v2];

    %the wheelchair geometric center predicted position is outside the
    %virtual box
    if robot_inside_obst==0
        alfa_12=V_12\VR';
    else
        alfa_12=[0;0];
    end

    %if the robot is in potential collision with the obstacle the constraint is computed,
    %otherwise no constraint is added
    if (robot_inside_obst==1 || (alfa_12(1)>0 && alfa_12(2)>0))
        [group(i_obs).hx, group(i_obs).hy, group(i_obs).l, ~]=constraintCoefficients_convex_hull(P1, P2, v_ped, VR, r_c, r_red, index, i_obs);
        plot(x_plot, -(group(i_obs).hx/group(i_obs).hy)*x_plot + group(i_obs).l/group(i_obs).hy, 'Color','r');
    end

    plot(group(i_obs).Q1(1), group(i_obs).Q1(2),'p', 'Color','r');
    plot(group(i_obs).Q2(1), group(i_obs).Q2(2),'o', 'Color','g');
end

plot(x_pr,y_pr);
plot(xunit, yunit,'LineStyle','--','Color',[1, 0.41, 0.16],'LineWidth',1.2,'DisplayName','Sensor Range'); % plotting the sensor range
scatter(x_pr(1),y_pr(1));
scatter(x_p0(1),y_p0(1),'*','b');
scatter(endLoc(1),endLoc(2),'*','b');
scatter(x,y,'g');
scatter(x_p,y_p,'r');
pause(0.1);
axis([-10 20 -10 20])
hold off

set(gcf, 'WindowState', 'maximized');
end

== matlab function wheelchair_navigation/Wheelchair dynamics /Wheelchair dynamics  ==
  data: v input; xdot output; omega input; theta input; ydot output; thdot output
function [xdot,ydot,thdot] = wheelchair_dynamics(v,omega,theta)

xdot  = v*cos(theta);
ydot  = v*sin(theta);
thdot = omega;

end

== matlab function wheelchair_navigation/MPC controller/MPC ==
  data: v_px output size=1; x_p input; y_p input; v_py output size=1; pose output; linear_position output; U_sl output; H_obs output; L_obs output; dl output; Ts parameter; N parameter; v_max parameter; q parameter; r parameter; a_max parameter; d parameter; Rw parameter; omega_m parameter; omega_M parameter; Usl_prev input; csi_prev input; curr_pose input; curr_ped_pos input; sp parameter; x_pr input; y_pr input; epsilon parameter; n_obs parameter; sa parameter; r_c parameter; r_red parameter; s parameter; opt_stat output; csi output; v_ped input; T_gp parameter; error output; replanTrigger input; param parameter; e parameter; N_samples parameter
function [v_px,v_py,pose,linear_position,U_sl,H_obs,L_obs,dl, opt_stat,csi, error] = MPC(x_p, y_p, Ts, N, v_max, q, r, a_max, d, Rw, omega_m,...
    omega_M, Usl_prev, csi_prev, curr_pose, curr_ped_pos, sp, x_pr,y_pr, epsilon, n_obs, sa, r_c, r_red, s, v_ped, T_gp, replanTrigger, param, e, N_samples)
%#codegen
coder.extrinsic('MPC_Controller');

%Initialization of vectors containing pedestrians predicted motion
current_x_ped = zeros(n_obs,1);
current_y_ped = zeros(n_obs,1);

%Position of pedestrians (obstacle) within the prediction horizon
current_x_ped(1:n_obs,1)=curr_ped_pos(1:n_obs);
current_y_ped(1:n_obs,1)=curr_ped_pos(n_obs+1:end);

X_ped = [current_x_ped, current_y_ped];


idx = dbscan(X_ped,2.7,1);

n_groups = max(idx);

n_groups_max = 100;

v_px=0; v_py=0;
error = 0;
pose=zeros(N,3); linear_position=zeros(N,2); csi=[0;0];
U_sl=zeros(2*N+n_groups_max+2,1);
H_obs=zeros(N,2*N,n_groups_max); L_obs=zeros(N,n_groups_max); dl=zeros(N,n_groups_max);
opt_stat = zeros(2,1);

[v_px,v_py,pose,linear_position,U_sl(1:2*N+n_groups+2,:),H_obs(:,:,1:n_groups),L_obs(:,1:n_groups),dl(:,1:n_groups), opt_stat, csi, error] = MPC_Controller(x_p, y_p, Ts, N, v_max, q, r, s, a_max, d, Rw, omega_m,...
    omega_M, Usl_prev, csi_prev, curr_pose, curr_ped_pos, v_ped, sp, x_pr, y_pr, epsilon, n_obs, sa, r_c, r_red, T_gp, replanTrigger, param, e, N_samples);


end

== matlab function wheelchair_navigation/pedestrianMotion/initialPosition ==
  data: Ped_init input; x_init output; y_init output; n_obs parameter
function [x_init,y_init] = initialPosition(Ped_init,n_obs)

x_init=Ped_init(1:n_obs,1);
y_init=Ped_init(1:n_obs,2);

end

== matlab function wheelchair_navigation/pedestrianMotion/pedestrianMotion ==
  data: xd_ped output; yd_ped output; n_obs parameter; v_ped input; theta_ped output
function [xd_ped,yd_ped,theta_ped]= pedestrianMotion(n_obs, v_ped)
    qd_ped=zeros(n_obs,2);
    xd_ped=zeros(n_obs,1);
    yd_ped=zeros(n_obs,1);
    theta_ped = zeros(n_obs,1);

    for i_obs=1:n_obs
        qd_ped(i_obs,1)=v_ped(i_obs,1);
        qd_ped(i_obs,2)=v_ped(i_obs,2);
        xd_ped(i_obs)=qd_ped(i_obs,1);
        yd_ped(i_obs)=qd_ped(i_obs,2);
        theta_ped(i_obs) = atan2(yd_ped(i_obs),xd_ped(i_obs));
    end
end

== matlab function wheelchair_navigation/Global  planner/Global Planner ==
  data: P_position input; x_pr output size=1,400; pedestrianData input; y_pr output size=1,400; current_time input; N parameter; n_obs parameter; v_ped parameter; endLoc parameter; Ts parameter; v_max parameter; a_max parameter; r_c parameter; T_gp parameter; replanningFlag input; y_pri parameter; x_pri parameter; v input; v_ref output size=1,400; a_ref output size=1,400; qd parameter; qdd parameter
function [x_pr, y_pr, v_ref, a_ref] = GlobalPlanner(P_position, pedestrianData, current_time, N, n_obs, v_ped, endLoc, Ts, v_max, ...
    a_max, r_c, T_gp, replanningFlag, y_pri, x_pri, v,qd, qdd)
    
    %#codegen
    coder.extrinsic('RRTXmain', 'trajectoryGeneration');
    coder.varsize('x_prev', 'y_prev', 'v_r', 'a_r');
    persistent x_prev
    persistent y_prev
    persistent v_r 
    persistent a_r

    % Obstacle vectors initialization
    x_ped=zeros(n_obs,N);
    y_ped=zeros(n_obs,N);

    % At initialization phase, the pedestrian path is simply its initial
    % position.
    if (isempty(x_prev))
        x_prev = x_pri;
        y_prev = y_pri;
        v_r = qd;
        a_r = qdd;
    end
    





    %Path generation and extraction --> If replanningFlag is false, the
    %robot trajectory doesnt change. Otherwise the RRTx algorithm is
    %activated and a new trajectory is computed
    x_pr = x_prev;
    y_pr = y_prev;
    v_ref = v_r;
    a_ref = a_r;
    if current_time > 1e-16 %workaround to align the code to the sampling time of the simulation
        startLoc = P_position';
        x_ped(1:n_obs,1) = pedestrianData(1:n_obs);
        y_ped(1:n_obs,1) = pedestrianData(n_obs+1:end);
        for i=2:N
            x_ped(:,i)=x_ped(:,i-1)+Ts*v_ped(:,1);
            y_ped(:,i)=y_ped(:,i-1)+Ts*v_ped(:,2);
        end
        path_ped = [x_ped' y_ped'];
    
        if (replanningFlag)
            % Find path for the wheelchair
            
            [graphTree, node, path_x, path_y, ~, path_graph, ~, ~] = RRTXmain(path_ped, r_c, Ts,startLoc, ...
            endLoc, v_ped, n_obs, N, false, current_time, replanningFlag);
            [x_pr, y_pr, v_ref, a_ref, ~] = trajectoryGeneration(path_x, path_y, v_max, a_max,Ts, v);
            x_prev = x_pr;
            y_prev = y_pr;
            v_r = v_ref; 
            a_r = a_ref;
                
        end
    end
    
end

== matlab function wheelchair_navigation/MPC controller/MATLAB Function ==
  data: pose_gt input; v input; omega input; qt input; pose output; param input; delta_prev input; delta output; mode_prev input; mode output; lost_idx_prev input; lost_idx output
function [pose,delta,mode,lost_idx] = AMCL(pose_gt,v,omega,qt,param,delta_prev,mode_prev,lost_idx_prev)

persistent jump_radius
persistent jump_angle

if isempty(jump_radius)
    jump_radius = 0;
end
if isempty(jump_angle)
    jump_angle = 0;
end

% Unroll parameters
rho            = param(1);
m_pos          = param(2);
q_pos          = param(3);
m_theta        = param(4);
q_theta        = param(5);
sigma_min_fact = param(6);
sigma_max_fact = param(7);
p_fail         = param(8);
lost_duration  = param(9);
qt_lost_thd    = param(10);
max_jump_dist  = param(11);

% Handle failure mode (1=tracking, 0=lost)
if (mode_prev==1) 
    if (qt<=qt_lost_thd) && (rand<=p_fail)
        mode = 0;
        lost_idx = 1;
        
        jump_radius = rand*max_jump_dist;
        jump_angle  = rand*2*pi;
    else
        mode = 1;
        lost_idx = 1;
    end
else
    if (qt>qt_lost_thd)
        mode = 1;
        lost_idx = 1;
    elseif (lost_idx_prev<=lost_duration)
        mode = 0;
        lost_idx = lost_idx_prev+1;
    else
        mode = 1;
        lost_idx = 1;
    end
end

% Compute noise standard deviation
sigma_pos   = m_pos*abs(v)+q_pos;
sigma_theta = m_theta*abs(omega)+q_theta;

% Apply scaling for perception quality
sigma_pos   = sigma_min_fact*sigma_pos+(1-qt)*(sigma_max_fact-sigma_min_fact)*sigma_pos;
sigma_theta = sigma_min_fact*sigma_theta+(1-qt)*(sigma_max_fact-sigma_min_fact)*sigma_theta;

% Noise correlation model
delta = rho*delta_prev+diag([sigma_pos,sigma_pos,sigma_theta])*randn(3,1);

% Localization data computation
pose = zeros(3,1);
if (mode==1)
    pose(1) = pose_gt(1)+cos(pose_gt(3))*delta(1)-sin(pose_gt(3))*delta(2);
    pose(2) = pose_gt(2)+sin(pose_gt(3))*delta(1)+cos(pose_gt(3))*delta(2);
    pose(3) = wrapToPi(pose_gt(3)+delta(3));
else
    pose_wr = zeros(3,1);
    pose_wr(1) = pose_gt(1)+jump_radius*cos(jump_angle);
    pose_wr(2) = pose_gt(2)+jump_radius*sin(jump_angle);
    pose_wr(3) = pose_gt(3);

    pose(1) = pose_wr(1)+cos(pose_wr(3))*delta(1)-sin(pose_wr(3))*delta(2);
    pose(2) = pose_wr(2)+sin(pose_wr(3))*delta(1)+cos(pose_wr(3))*delta(2);
    pose(3) = wrapToPi(pose_wr(3)+delta(3));
end

== matlab function wheelchair_navigation/MPC controller/point P kinematics ==
  data: x input; x_p output; y input; theta input; y_p output; epsilon parameter
function [x_p,y_p] = pointKinematics(x,y,theta,epsilon)

    
    x_p = x+epsilon*cos(theta);
    y_p = y+epsilon*sin(theta);

end

== matlab function wheelchair_navigation/Pedestrian estimator/Pedestrian position estimation (1 pedestrian)/MATLAB Function ==
  data: ped_pose_gt input; ped_pos output size=2; robot_pos_gt_x input; robot_pos_gt_y input; param input
function ped_pos = measured_ped_pos(ped_pose_gt,robot_pos_gt_x,robot_pos_gt_y,param)

% Pedestrian position (actual and ground trut)
% x_1, x_2, ..., x_n_obs, y_1, y_2, ..., y_n_obs

n_obs = 1; % Set output size accordingly in edit data

% Unroll parameters
sigma_q = param(1);
sigma_m = param(2);

robot_pos_gt = [robot_pos_gt_x,robot_pos_gt_y];

% Compute estimated pedestrian positions
ped_pos = zeros(2*n_obs,1);
for k=1:n_obs
    % k-th pedestrian pose
    pedk_pose_gt = [ped_pose_gt(k), ped_pose_gt(k+n_obs), ped_pose_gt(k+2*n_obs)];

    % Noise variance
    sigma = sigma_q+sigma_m*norm(robot_pos_gt-pedk_pose_gt(1:2));

    % Position estimate
    delta = randn*sigma;
    ped_pos(k)       = pedk_pose_gt(1)+cos(pedk_pose_gt(3))*delta-sin(pedk_pose_gt(3))*delta;
    ped_pos(k+n_obs) = pedk_pose_gt(2)+sin(pedk_pose_gt(3))*delta+cos(pedk_pose_gt(3))*delta;
end

== matlab function wheelchair_navigation/Pedestrian estimator/Pedestrian position estimation (4 pedestrians)/MATLAB Function ==
  data: ped_pose_gt input; ped_pos output size=8; robot_pos_gt_x input; robot_pos_gt_y input; param input
function ped_pos = measured_ped_pos(ped_pose_gt,robot_pos_gt_x,robot_pos_gt_y,param)

% Pedestrian position (actual and ground trut)
% x_1, x_2, ..., x_n_obs, y_1, y_2, ..., y_n_obs

n_obs = 4; % Set output size accordingly in edit data

% Unroll parameters
sigma_q = param(1);
sigma_m = param(2);

robot_pos_gt = [robot_pos_gt_x,robot_pos_gt_y];

% Compute estimated pedestrian positions
ped_pos = zeros(2*n_obs,1);
for k=1:n_obs
    % k-th pedestrian pose
    pedk_pose_gt = [ped_pose_gt(k), ped_pose_gt(k+n_obs), ped_pose_gt(k+2*n_obs)];

    % Noise variance
    sigma = sigma_q+sigma_m*norm(robot_pos_gt-pedk_pose_gt(1:2));

    % Position estimate
    delta = randn*sigma;
    ped_pos(k)       = pedk_pose_gt(1)+cos(pedk_pose_gt(3))*delta-sin(pedk_pose_gt(3))*delta;
    ped_pos(k+n_obs) = pedk_pose_gt(2)+sin(pedk_pose_gt(3))*delta+cos(pedk_pose_gt(3))*delta;
end

== matlab function wheelchair_navigation/Pedestrian estimator/Pedestrian position estimation (6 pedestrians)1/MATLAB Function ==
  data: ped_pose_gt input; ped_pos output size=12; robot_pos_gt_x input; robot_pos_gt_y input; param input
function ped_pos = measured_ped_pos(ped_pose_gt,robot_pos_gt_x,robot_pos_gt_y,param)

% Pedestrian position (actual and ground trut)
% x_1, x_2, ..., x_n_obs, y_1, y_2, ..., y_n_obs

n_obs = 6; % Set output size accordingly in edit data

% Unroll parameters
sigma_q = param(1);
sigma_m = param(2);

robot_pos_gt = [robot_pos_gt_x,robot_pos_gt_y];

% Compute estimated pedestrian positions
ped_pos = zeros(2*n_obs,1);
for k=1:n_obs
    % k-th pedestrian pose
    pedk_pose_gt = [ped_pose_gt(k), ped_pose_gt(k+n_obs), ped_pose_gt(k+2*n_obs)];

    % Noise variance
    sigma = sigma_q+sigma_m*norm(robot_pos_gt-pedk_pose_gt(1:2));

    % Position estimate
    delta = randn*sigma;
    ped_pos(k)       = pedk_pose_gt(1)+cos(pedk_pose_gt(3))*delta-sin(pedk_pose_gt(3))*delta;
    ped_pos(k+n_obs) = pedk_pose_gt(2)+sin(pedk_pose_gt(3))*delta+cos(pedk_pose_gt(3))*delta;
end
